simulink model "Q1"  (R2018a)
settings: Solver=VariableStepAuto  StartTime=0.0  StopTime=1e5  RelTol=1e-3
undefined symbols (not defined in the file or in its folder): m, n
settings Model: SimulationMode=accelerator  Creator=Mohamed Saber  LastModifiedBy=Mohamed Saber

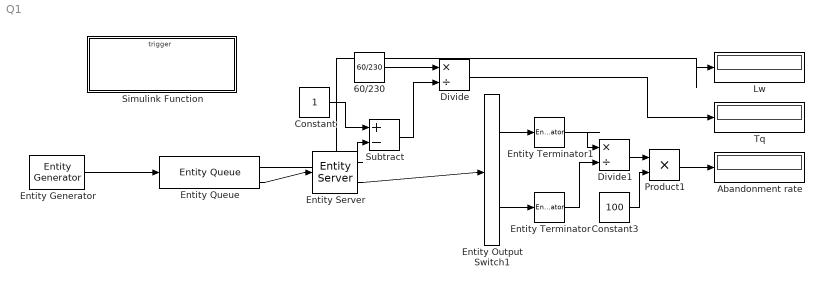
== system Q1 ==
  60/230 : Constant  Value=60/230
  Abandonment rate : Display
  Constant : Constant
  Constant3 : Constant  Value=100
  Divide : Product  Inputs=*/
  Divide1 : Product  Inputs=*/
  Entity Output Switch1 : EntityOutputSwitch  InputPortMessageModes=m  OutputPortMessageModes=m,m  SwitchingCriterion=From attribute  SwitchAttributeName=Exit
  Entity Generator : EntityGenerator  OutputPortMessageModes=m  TimeSource=MATLAB action  IntergenerationTimeAction=|  GenerateAction=|  AttributeName=ClassA|Impatient|StartTime|Exit  AttributeInitialValue=1|1|0|2  EntityType=Structured  EntityTypeName=Entity
      IntergenerationTimeAction=|
      | dt = rand(1,1);
      | persistent rngInit;
      | if isempty(rngInit)
      |     seed = 12345;
      |     rng(seed);
      |     rngInit = true;
      | end
      | 
      | % Pattern: Exponential distribution
      | mu = 60/220;
      | dt = -mu * log(1 - rand());
      GenerateAction=|
      | persistent rngInit;
      | if isempty(rngInit)
      |     seed = 15318;
      |     rng(seed);
      |     rngInit = true;
      | end
      | 
      | % Pattern: Arbitrary discrete distribution
      | % V: Value vector
      | % P: Probability vector
      | V = [1 2];
      | P = [0.2 0.8];
      | entity.ClassA = randsample(V, 1, true, P);
      | 
      | % Pattern: Arbitrary discrete distribution
      | % V: Value vector
      | % P: Probability vector
      | V = [1 2];
      | P = [0.1 0.9];
      | entity.Impatient = randsample(V, 1, true, P);
      | 
      | entity.StartTime = getCurrentTime();
  Entity Queue : EntityQueue  InputPortMessageModes=m  OutputPortMessageModes=n,m  Capacity=inf  QueueType=Priority  PrioritySource=ClassA  AverageQueueLength=on
      settings: OutputPortMap=o3,o5
  Entity Server : EntityServer  InputPortMessageModes=m  OutputPortMessageModes=n,m  Capacity=1  ServiceTimeSource=MATLAB action  ServiceTimeValue=60/220  ServiceTimeAttributeName=ClassA  ServiceTimeAction=|  EntryAction=|  Utilization=on
      ServiceTimeAction=|
      | dt = rand(1,1);
      | persistent rngInit;
      | if isempty(rngInit)
      |     seed = 845889;
      |     rng(seed);
      |     rngInit = true;
      | end
      | 
      | % Pattern: Exponential distribution
      | mu = 60/230;
      | dt = -mu * log(1 - rand());
      EntryAction=|
      | TimeTaken = (getCurrentTime()-entity.StartTime);
      | if entity.Impatient ==1 && TimeTaken>3
      |     entity.Exit=1;
      | end
      settings: OutputPortMap=o5,o9
  Entity Terminator : EntityTerminator  InputPortMessageModes=m  NumberEntitiesArrived=on
      settings: OutputPortMap=o0
  Entity Terminator1 : EntityTerminator  InputPortMessageModes=m  NumberEntitiesArrived=on
      settings: OutputPortMap=o0
  Lw : Display
      settings: Format=bank  Decimation=5
  Product1 : Product
  Simulink Function : Subsystem  TreatAsAtomicUnit=on
  Subtract : Sum  Inputs=+-
  Tq : Display
  wires:
  Divide/1 -> Tq/1
  Entity Terminator/1 -> Divide1/2
  Divide1/1 -> Product1/1
  Entity Terminator1/1 -> Divide1/1
  Constant3/1 -> Product1/2
  Subtract/1 -> Divide/2
  Entity Queue/1 -> Lw/1
  Entity Server/1 -> Subtract/2
  60/230/1 -> Divide/1
  Product1/1 -> Abandonment rate/1
  Entity Output Switch1/1 -> Entity Terminator1/1
  Entity Generator/1 -> Entity Queue/1
  Constant/1 -> Subtract/1
  Entity Queue/2 -> Entity Server/1
  Entity Output Switch1/2 -> Entity Terminator/1
  Entity Server/2 -> Entity Output Switch1/1

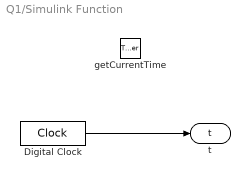
== system Q1/Simulink Function ==
  getCurrentTime : TriggerPort  TriggerType=function-call  IsSimulinkFunction=on  FunctionName=getCurrentTime  VariantControl=(inherit)
  Digital Clock : DigitalClock  SampleTime=-1
  t : ArgOut  DisableCoverage=on  ArgumentName=t
  wires:
  Digital Clock/1 -> t/1
